simulink model "sampleModel1856"  (R2023a)
settings: Solver=VariableStepAuto  StartTime=0.0  StopTime=10.0  RelTol=1e-3
libraries: simulink x5, hdlsllib x4
settings Model: Creator=user1  LastModifiedBy=user1

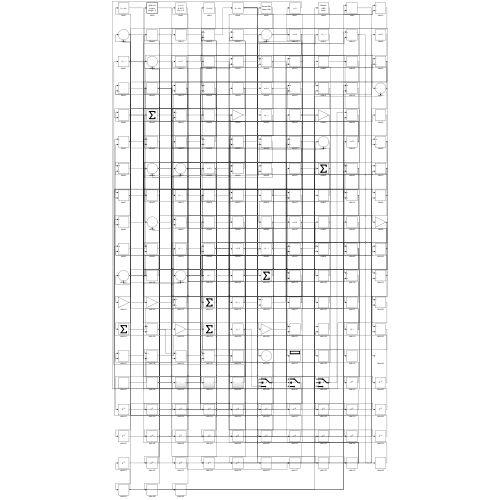
[thumbnail: Simulink's stored preview of the top-level diagram]
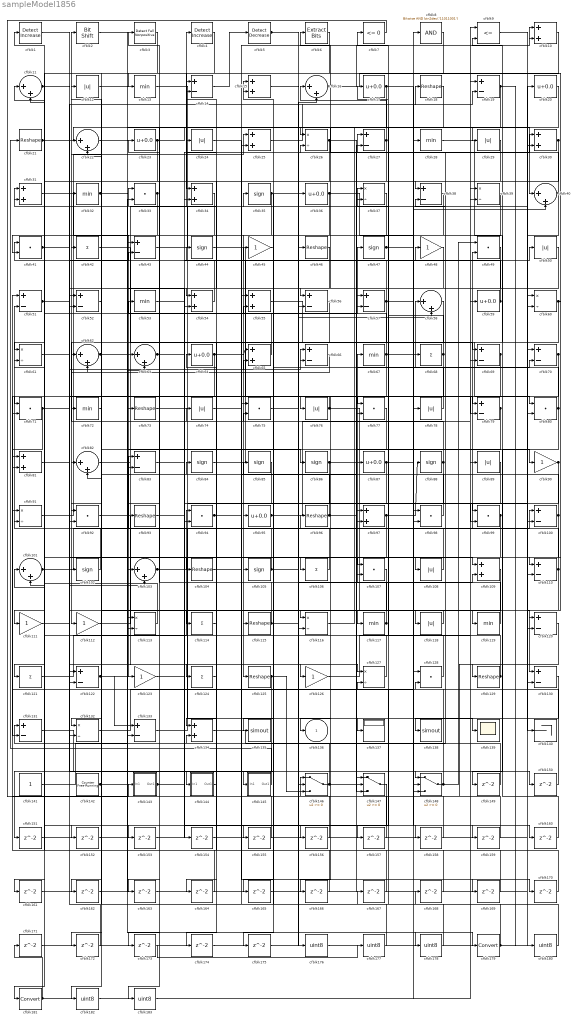
== system sampleModel1856 ==
  cfblk1 : simulink/Logic and Bit Operations/Detect Increase  vinit=0.0  OutDataTypeStr=boolean
      settings: LibrarySourceBlock=|
      | hdlsllib/Logic and Bit
      | Operations/Detect
      | Increase
  cfblk{10,15,25,30..31,34,54..55,65,81,97,109,134} (13 alike) : Sum
  cfblk{14,19,27,38,43,51..52,56..57,66,69..70,79,83,100,110,120,122,130..131,133} (21 alike) : Sum  Inputs=+-
  cfblk{11,16,22,40,58,62..63,82,101,103} (10 alike) : Sum  Inputs=|++
  cfblk{35,44,47,84..86,88,102,105} (9 alike) : Signum
  cfblk{18,21,46,73,93,96,104,115,125,129} (10 alike) : Reshape
  cfblk{42,68,106,114,121,124} (6 alike) : Sum  Inputs=+
  cfblk{33,41,49,71,75,77,80,92,94,98..99,107,128} (13 alike) : DotProduct  OutDataTypeStr=Inherit: Inherit via internal rule
  cfblk{12,24,29,50,74,76,78,89,108,118} (10 alike) : Abs  SaturateOnIntegerOverflow=off
  cfblk{45,48,90,111..112,123,126} (7 alike) : Gain
  cfblk{26,37,39,60..61,91,113,116,127,132} (10 alike) : Product  Inputs=*/  RndMeth=Zero  SaturateOnIntegerOverflow=on
  cfblk{13,28,32,53,67,72,117,119} (8 alike) : MinMax
  cfblk135 : ToWorkspace  VariableName=simout  SaveFormat=Timeseries  SampleTime=-1
  cfblk137 : Display
  cfblk138 : ToWorkspace  VariableName=simout  SaveFormat=Timeseries  SampleTime=-1
  cfblk139 : Scope
  cfblk140 : Terminator
  cfblk141 : Constant  SampleTime=-1
  cfblk142 : hdlsllib/Sources/Counter Free-Running  NumBits=16  tsamp=-1
  cfblk143 : Subsystem
      settings: LibrarySourceBlock=|
      | hdlsllib/Ports &
      | Subsystems/Subsystem
  cfblk144 : Subsystem
      settings: LibrarySourceBlock=|
      | hdlsllib/Ports &
      | Subsystems/Subsystem
  cfblk145 : Subsystem
      settings: LibrarySourceBlock=|
      | hdlsllib/Ports &
      | Subsystems/Subsystem
  cfblk146 : Switch  SaturateOnIntegerOverflow=off  InputSameDT=off
  cfblk147 : Switch  SaturateOnIntegerOverflow=off  InputSameDT=off
  cfblk148 : Switch  SaturateOnIntegerOverflow=off  InputSameDT=off
  cfblk{149..175} (27 alike) : Delay  SampleTime=1
  cfblk{17,20,23,36,59,64,87,95} (8 alike) : Bias  Bias=0.0  SaturateOnIntegerOverflow=off
  cfblk{176..178,180,182..183} (6 alike) : DataTypeConversion  OutDataTypeStr=uint8  SaturateOnIntegerOverflow=off  RndMeth=Floor
  cfblk179 : DataTypeConversion  SaturateOnIntegerOverflow=off  RndMeth=Floor
  cfblk181 : DataTypeConversion  SaturateOnIntegerOverflow=off  RndMeth=Floor
  cfblk2 : hdlsllib/Logic and Bit Operations/Bit Shift  mode=Shift Left Logical  N=0
  cfblk3 : hdlsllib/Logic and Bit Operations/Detect Fall Nonpositive  vinit=0  OutDataTypeStr=boolean
  cfblk4 : simulink/Logic and Bit Operations/Detect Increase  vinit=0.0  OutDataTypeStr=boolean
      settings: LibrarySourceBlock=|
      | hdlsllib/Logic and Bit
      | Operations/Detect
      | Increase
  cfblk5 : simulink/Logic and Bit Operations/Detect Decrease  vinit=0.0  OutDataTypeStr=boolean
      settings: LibrarySourceBlock=|
      | hdlsllib/Logic and Bit
      | Operations/Detect
      | Decrease
  cfblk6 : simulink/Logic and Bit Operations/Extract Bits  bitsToExtract=Upper half  numBits=8  bitIdxRange=[0 7]  outScalingMode=Preserve fixed-point scaling
      settings: LibrarySourceBlock=|
      | hdlsllib/Logic and Bit
      | Operations/Extract Bits
  cfblk7 : hdlsllib/Logic and Bit Operations/Compare To Zero  relop=<=  OutDataTypeStr=boolean
  cfblk8 : simulink/Logic and Bit Operations/Bitwise Operator  logicop=AND  UseBitMask=on  BitMask=bin2dec('11011001')  BitMaskRealWorld=Stored Integer
      settings: LibrarySourceBlock=|
      | hdlsllib/Logic and Bit
      | Operations/Bitwise
      | Operator
  cfblk9 : RelationalOperator  Operator=<=  OutDataTypeStr=boolean  InputSameDT=off
  cfblk136 : Outport  VectorParamsAs1DForOutWhenUnconnected=off
  wires:
  cfblk73/1 -> cfblk137/1
  cfblk128/1 -> cfblk33/1
  cfblk117/1 -> cfblk67/1, cfblk31/1
  cfblk148/1 -> cfblk49/1, cfblk128/2
  cfblk134/1 -> cfblk27/1
  cfblk116/1 -> cfblk40/1
  cfblk146/1 -> cfblk131/1, cfblk150/1
  cfblk69/1 -> cfblk81/2, cfblk152/1
  cfblk49/1 -> cfblk125/1
  cfblk18/1 -> cfblk117/1
  cfblk92/1 -> cfblk126/1
  cfblk28/1 -> cfblk80/1
  cfblk84/1 -> cfblk48/1
  cfblk27/1 -> cfblk16/1, cfblk83/2
  cfblk67/1 -> cfblk47/1, cfblk136/1, cfblk82/2, cfblk31/2, cfblk160/1
  cfblk120/1 -> cfblk146/1
  cfblk130/1 -> cfblk138/1
  cfblk91/1 -> cfblk25/1
  cfblk33/1 -> cfblk123/1, cfblk101/2
  cfblk88/1 -> cfblk2/1, cfblk156/1
  cfblk78/1 -> cfblk58/1
  cfblk16/1 -> cfblk110/1, cfblk10/1
  cfblk145/1(Out1) -> cfblk21/1
  cfblk26/1 -> cfblk90/1, cfblk163/1
  cfblk56/1 -> cfblk112/1
  cfblk105/1 -> cfblk51/2, cfblk109/1, cfblk109/2
  cfblk4/1 -> cfblk121/1
  cfblk121/1 -> cfblk94/1
  cfblk131/1 -> cfblk144/1(In1)
  cfblk112/1 -> cfblk4/1
  cfblk6/1 -> cfblk146/2
  cfblk80/1 -> cfblk15/1, cfblk149/1
  cfblk96/1 -> cfblk3/1, cfblk148/3
  cfblk58/1 -> cfblk82/1
  cfblk9/1 -> cfblk60/2
  cfblk108/1 -> cfblk17/1
  cfblk13/1 -> cfblk140/1
  cfblk31/1 -> cfblk43/1
  cfblk45/1 -> cfblk15/2
  cfblk132/1 -> cfblk28/1
  cfblk14/1 -> cfblk5/1
  cfblk68/1 -> cfblk37/1, cfblk166/1
  cfblk21/1 -> cfblk29/1, cfblk147/2
  cfblk52/1 -> cfblk92/1
  cfblk102/1 -> cfblk11/1
  cfblk10/1 -> cfblk13/1
  cfblk8/1 -> cfblk34/1
  cfblk17/1 -> cfblk63/1, cfblk100/2, cfblk56/1
  cfblk118/1 -> cfblk116/1
  cfblk89/1 -> cfblk94/2
  cfblk11/1 -> cfblk61/1, cfblk79/2
  cfblk39/1 -> cfblk181/1
  cfblk62/1 -> cfblk76/1, cfblk104/1
  cfblk44/1 -> cfblk77/1
  cfblk63/1 -> cfblk119/1, cfblk50/1, cfblk155/1
  cfblk43/1 -> cfblk20/1
  cfblk54/1 -> cfblk41/1
  cfblk47/1 -> cfblk40/2, cfblk159/1
  cfblk76/1 -> cfblk130/1, cfblk73/1
  cfblk85/1 -> cfblk115/1
  cfblk81/1 -> cfblk66/1
  cfblk133/1 -> cfblk49/2
  cfblk119/1 -> cfblk23/1
  cfblk37/1 -> cfblk95/1
  cfblk55/1 -> cfblk69/1
  cfblk65/1 -> cfblk42/1
  cfblk64/1 -> cfblk65/1, cfblk71/2
  cfblk143/1(Out1) -> cfblk30/1, cfblk37/2
  cfblk97/1 -> cfblk88/1, cfblk111/1
  cfblk3/1 -> cfblk72/1
  cfblk115/1 -> cfblk97/1, cfblk53/1
  cfblk122/1 -> cfblk133/1, cfblk55/2
  cfblk42/1 -> cfblk147/1
  cfblk46/1 -> cfblk135/1
  cfblk125/1 -> cfblk45/1, cfblk146/3, cfblk151/1
  cfblk1/1 -> cfblk124/1
  cfblk82/1 -> cfblk65/2
  cfblk36/1 -> cfblk92/2, cfblk78/1
  cfblk141/1 -> cfblk33/2
  cfblk41/1 -> cfblk118/1, cfblk103/2
  cfblk35/1 -> cfblk36/1, cfblk41/2, cfblk175/1
  cfblk101/1 -> cfblk108/1, cfblk56/2
  cfblk30/1 -> cfblk38/1, cfblk52/2
  cfblk144/1(Out1) -> cfblk84/1
  cfblk126/1 -> cfblk59/1
  cfblk2/1 -> cfblk116/2
  cfblk19/1 -> cfblk133/2, cfblk180/1
  cfblk129/1 -> cfblk97/2, cfblk38/2
  cfblk127/1 -> cfblk61/2
  cfblk93/1 -> cfblk105/1
  cfblk142/1 -> cfblk63/2, cfblk96/1, cfblk22/2
  cfblk95/1 -> cfblk19/1, cfblk19/2
  cfblk7/1 -> cfblk143/1(In1)
  cfblk106/1 -> cfblk83/1
  cfblk83/1 -> cfblk35/1
  cfblk57/1 -> cfblk132/1, cfblk93/1, cfblk32/1, cfblk99/1
  cfblk61/1 -> cfblk18/1
  cfblk59/1 -> cfblk24/1, cfblk44/1
  cfblk104/1 -> cfblk87/1
  cfblk23/1 -> cfblk71/1, cfblk26/1
  cfblk90/1 -> cfblk99/2, cfblk164/1
  cfblk29/1 -> cfblk54/1
  cfblk66/1 -> cfblk62/2
  cfblk38/1 -> cfblk77/2
  cfblk98/1 -> cfblk7/1
  cfblk103/1 -> cfblk100/1, cfblk80/2, cfblk26/2
  cfblk25/1 -> cfblk9/1
  cfblk79/1 -> cfblk147/3, cfblk162/1
  cfblk12/1 -> cfblk179/1
  cfblk22/1 -> cfblk79/1
  cfblk114/1 -> cfblk64/1
  cfblk100/1 -> cfblk85/1, cfblk129/1, cfblk102/1, cfblk22/1
  cfblk32/1 -> cfblk86/1, cfblk114/1, cfblk54/2
  cfblk70/1 -> cfblk106/1, cfblk66/2
  cfblk48/1 -> cfblk132/2
  cfblk86/1 -> cfblk70/2, cfblk145/1(In1)
  cfblk60/1 -> cfblk134/1, cfblk120/1
  cfblk113/1 -> cfblk91/2
  cfblk111/1 -> cfblk43/2
  cfblk15/1 -> cfblk46/1
  cfblk110/1 -> cfblk130/2, cfblk74/1
  cfblk74/1 -> cfblk57/1
  cfblk40/1 -> cfblk6/1, cfblk120/2
  cfblk24/1 -> cfblk148/1
  cfblk99/1 -> cfblk107/1, cfblk165/1, cfblk183/1
  cfblk94/1 -> cfblk10/2, cfblk169/1, cfblk170/1
  cfblk34/1 -> cfblk113/2
  cfblk124/1 -> cfblk14/1
  cfblk87/1 -> cfblk98/2, cfblk107/2
  cfblk51/1 -> cfblk122/2, cfblk11/2
  cfblk71/1 -> cfblk103/1, cfblk131/2
  cfblk5/1 -> cfblk139/1, cfblk127/1, cfblk58/2, cfblk178/1
  cfblk149/1 -> cfblk134/2
  cfblk150/1 -> cfblk51/1
  cfblk151/1 -> cfblk34/2
  cfblk152/1 -> cfblk60/1
  cfblk77/1 -> cfblk153/1
  cfblk153/1 -> cfblk25/2
  cfblk123/1 -> cfblk154/1
  cfblk154/1 -> cfblk27/2
  cfblk155/1 -> cfblk62/1
  cfblk156/1 -> cfblk55/1
  cfblk20/1 -> cfblk157/1
  cfblk157/1 -> cfblk52/1
  cfblk53/1 -> cfblk158/1
  cfblk158/1 -> cfblk98/1
  cfblk159/1 -> cfblk81/1
  cfblk160/1 -> cfblk9/2
  cfblk147/1 -> cfblk161/1
  cfblk161/1 -> cfblk69/2
  cfblk162/1 -> cfblk113/1
  cfblk163/1 -> cfblk110/2
  cfblk164/1 -> cfblk91/1
  cfblk165/1 -> cfblk57/2
  cfblk166/1 -> cfblk101/1
  cfblk167/1 -> cfblk1/1
  cfblk168/1 -> cfblk128/1
  cfblk169/1 -> cfblk148/2
  cfblk170/1 -> cfblk14/2
  cfblk171/1 -> cfblk30/2
  cfblk107/1 -> cfblk172/1
  cfblk172/1 -> cfblk122/1
  cfblk50/1 -> cfblk173/1
  cfblk109/1 -> cfblk174/1
  cfblk174/1 -> cfblk16/2
  cfblk175/1 -> cfblk70/1
  cfblk75/1 -> cfblk176/1
  cfblk176/1 -> cfblk8/1
  cfblk173/1 -> cfblk177/1
  cfblk177/1 -> cfblk75/1
  cfblk178/1 -> cfblk75/2
  cfblk179/1 -> cfblk168/1, cfblk167/1, cfblk127/2
  cfblk180/1 -> cfblk12/1
  cfblk181/1 -> cfblk171/1, cfblk89/1, cfblk68/1
  cfblk72/1 -> cfblk182/1
  cfblk182/1 -> cfblk39/1
  cfblk183/1 -> cfblk39/2

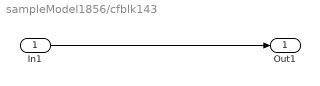
== system sampleModel1856/cfblk143 ==
  In1 : Inport
  Out1 : Outport
  wires:
  In1/1 -> Out1/1

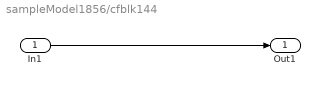
== system sampleModel1856/cfblk144 ==
  In1 : Inport
  Out1 : Outport
  wires:
  In1/1 -> Out1/1

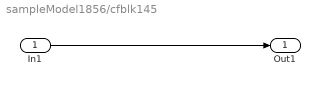
== system sampleModel1856/cfblk145 ==
  In1 : Inport
  Out1 : Outport
  wires:
  In1/1 -> Out1/1
